simulink model "PID_Control_Analysis"  (R2020b)
settings: Solver=VariableStepAuto  StartTime=0.0  StopTime=15  RelTol=1e-3  AbsTol=1e-3
model workspace (MAT data in the model file):
  Integral_Scale = 1
  Kd_percent = 49.9526515152
  Ki = 0.575757575758
  Km = 1
  Kp = 0.345454545455
  Proportional_Scale = 1
  R = 2
  Wn = 4
  sigma = 0.4
settings Model: OrderedModelArguments=off  Creator=callu  LastModifiedBy=callu
settings SolverCC: AutoScaleAbsTol=off  AlgebraicLoopSolver=LineSearch
settings DebuggingCC: SymbolicDimsDataTypeCodeGenerationDiagnostic=none
settings SFSimCC: CustomCodeUndefinedFunction=UseInterfaceOnly
settings SimscapeCC: SimscapeLogType=all  SimscapeLogSimulationStatistics=on  SimscapeLogDataHistory=10000

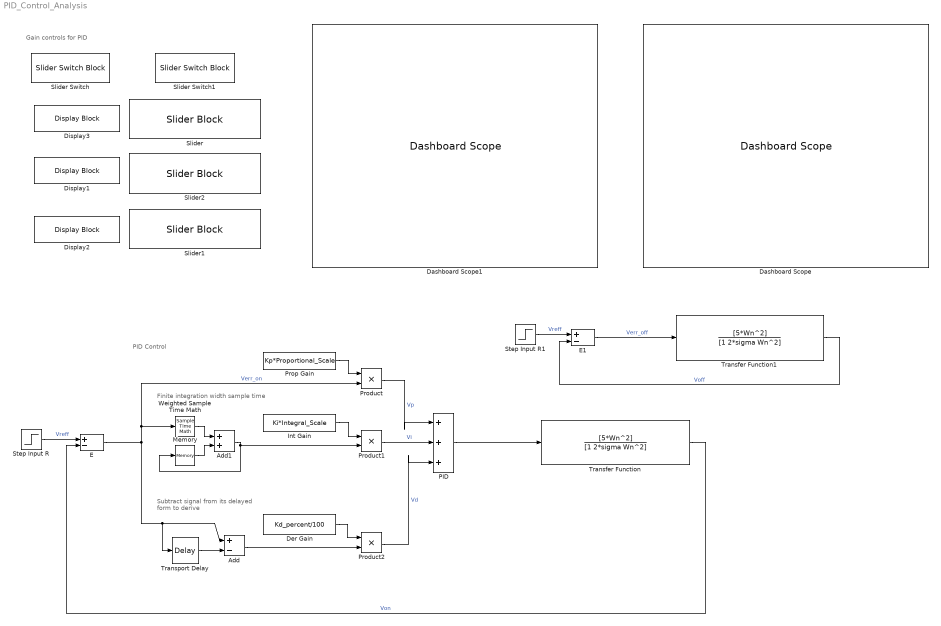
== system PID_Control_Analysis ==
  note: PID Control
  note: Gain controls for PID
  note: Subtract signal from its
      | delayed form to derive
  note: Finite integration
      | width sample time
  Add : Sum  Inputs=+-
  Add1 : Sum
  Dashboard Scope : DashboardScope
      settings: AttributesFormatString=System Response
  Dashboard Scope1 : DashboardScope
      settings: AttributesFormatString=PID Control Signals
  Der Gain : Constant  Value=Kd_percent/100
  Display1 : DisplayBlock  Format=short  Transparency=1
  Display2 : DisplayBlock  Format=short  Transparency=1
  Display3 : DisplayBlock  Format=short  Transparency=1
  E : Sum  Inputs=|+|-|
  E1 : Sum  Inputs=|+|-|
  Int Gain : Constant  Value=Ki*Integral_Scale
  Memory : Memory
  PID : Sum  Inputs=|+|+|+|
  Product : Product
  Product1 : Product
  Product2 : Product
  Prop Gain : Constant  Value=Kp*Proportional_Scale
  Slider : SliderBlock  ScaleMax=1  TickInterval=0.1
  Slider Switch : SliderSwitchBlock
      settings: Values={{'1', '10'}, [1 10]}
  Slider Switch1 : SliderSwitchBlock
      settings: Values={{'1', '10'}, [1 10]}
  Slider1 : SliderBlock  TickInterval=10
  Slider2 : SliderBlock  ScaleMax=1  TickInterval=0.1
  Step Input R : Step  After=R  SampleTime=0
  Step Input R1 : Step  After=R  SampleTime=0
  Transfer Function : TransferFcn  Numerator=[5*Wn^2]  Denominator=[1 2*sigma Wn^2]
  Transfer Function1 : TransferFcn  Numerator=[5*Wn^2]  Denominator=[1 2*sigma Wn^2]
  Transport Delay : TransportDelay  DelayTime=0.1
  Weighted Sample Time Math : SampleTimeMath  TsampMathOp=*
  wires:
  Step Input R/1 -> E/1  "Vreff"
  E/1 -> Transport Delay/1, Add/1, Product/2, Weighted Sample Time Math/1  "Verr_on"
  Transfer Function/1 -> E/2  "Von"
  PID/1 -> Transfer Function/1
  Transfer Function1/1 -> E1/2  "Voff"
  Step Input R1/1 -> E1/1  "Vreff"
  E1/1 -> Transfer Function1/1  "Verr_off"
  Add1/1 -> Memory/1, Product1/2
  Memory/1 -> Add1/2
  Weighted Sample Time Math/1 -> Add1/1
  Transport Delay/1 -> Add/2
  Product2/1 -> PID/3  "Vd"
  Product1/1 -> PID/2  "Vi"
  Prop Gain/1 -> Product/1
  Product/1 -> PID/1  "Vp"
  Der Gain/1 -> Product2/1
  Add/1 -> Product2/2
  Int Gain/1 -> Product1/1
